simulink model "model"  (R2021a)
settings: Solver=ode23s  StartTime=0.0  StopTime=0.04  MaxStep=1e-4  RelTol=1e-3
undefined symbols (not defined in the file): D1, L, lagging, pulse
libraries: spsACVoltageSourceLib x6, spsSeriesRLCBranchLib x6, spsGroundLib x5, spsThreePhaseTransformerTwoWindingsLib x4, spsUniversalBridgeLib x4, spsVoltageMeasurementLib x3, spsPulseGeneratorThyristor6PulseLib x2, simulink x2, spsControlledCurrentSourceLib x1, spsCurrentMeasurementLib x1, spsPower3phInstantaneousLib x1, spsThreePhaseVIMeasurementLib x1
settings Model: Creator=Tasneem  LastModifiedBy=Tasneem

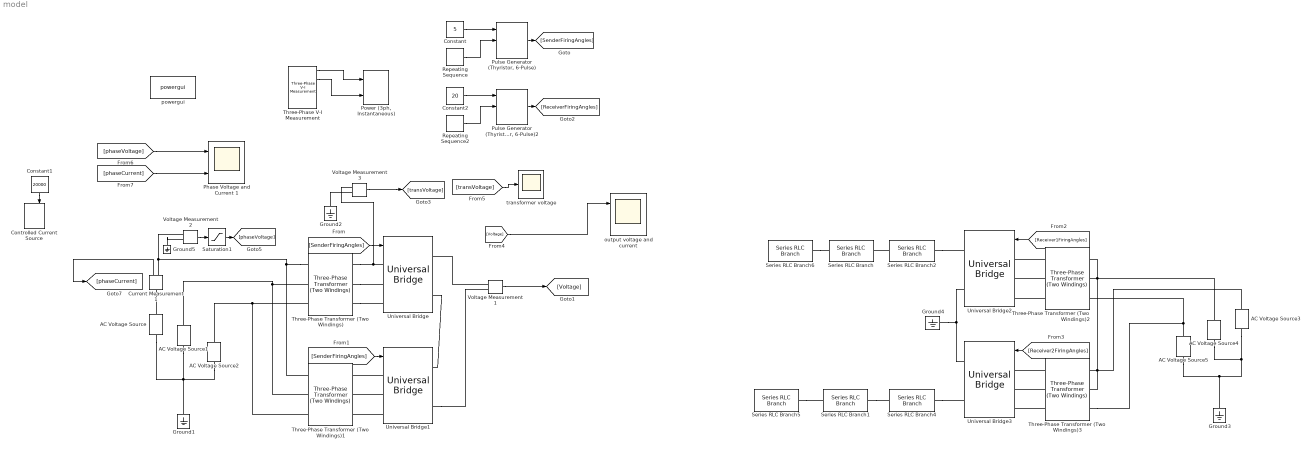
== system model ==
  AC Voltage Source : spsACVoltageSourceLib/AC Voltage Source  Amplitude=22e3  Phase=0  Frequency=50  SampleTime=0  Measurements=None  BusType=swing  Pref=10e3  Qref=0  Qmin=-inf  Qmax=+inf
  AC Voltage Source1 : spsACVoltageSourceLib/AC Voltage Source  Amplitude=22e3  Phase=-120  Frequency=50  SampleTime=0  Measurements=None  BusType=swing  Pref=10e3  Qref=0  Qmin=-inf  Qmax=+inf
  AC Voltage Source2 : spsACVoltageSourceLib/AC Voltage Source  Amplitude=22e3  Phase=120  Frequency=50  SampleTime=0  Measurements=None  BusType=swing  Pref=10e3  Qref=0  Qmin=-inf  Qmax=+inf
  AC Voltage Source3 : spsACVoltageSourceLib/AC Voltage Source  Amplitude=20000*sqrt(2/3)  Phase=0  Frequency=60  SampleTime=0  Measurements=None  BusType=swing  Pref=10e3  Qref=0  Qmin=-inf  Qmax=+inf
  AC Voltage Source4 : spsACVoltageSourceLib/AC Voltage Source  Amplitude=20000*sqrt(2/3)  Phase=-120  Frequency=60  SampleTime=0  Measurements=None  BusType=swing  Pref=10e3  Qref=0  Qmin=-inf  Qmax=+inf
  AC Voltage Source5 : spsACVoltageSourceLib/AC Voltage Source  Amplitude=20000*sqrt(2/3)  Phase=120  Frequency=60  SampleTime=0  Measurements=None  BusType=swing  Pref=10e3  Qref=0  Qmin=-inf  Qmax=+inf
  Constant : Constant  Value=5
  Constant1 : Constant  Value=20000
  Constant2 : Constant  Value=20
  Controlled Current Source : spsControlledCurrentSourceLib/Controlled Current Source  Initialize=on  Source_Type=AC  Amplitude=0  Phase=0  Frequency=0  Measurements=None
  Current Measurement1 : spsCurrentMeasurementLib/Current Measurement  PhasorSimulation=off  OutputType=Complex  PSBequivalent=0
  Ground{1..5} (5 alike) : spsGroundLib/Ground  LConnTagsString=a
  Phase Voltage and Current 1 : Scope  NumInputPorts=2
  "Power (3ph, Instantaneous)" : spsPower3phInstantaneousLib/Power (3ph, Instantaneous)
  "Pulse Generator (Thyristor, 6-Pulse)" : spsPulseGeneratorThyristor6PulseLib/Pulse Generator (Thyristor, 6-Pulse)  GenType=6-pulse  Delta=D1 (lagging)  pwidth=60  Double_Pulse=off  Ts=0
      settings: SourceProductBaseCode=PS
  "Pulse Generator (Thyristor, 6-Pulse)2" : spsPulseGeneratorThyristor6PulseLib/Pulse Generator (Thyristor, 6-Pulse)  GenType=6-pulse  Delta=D1 (lagging)  pwidth=60  Double_Pulse=off  Ts=0
      settings: SourceProductBaseCode=PS
  Repeating Sequence : simulink/Sources/Repeating Sequence  rep_seq_t=[0 1/50]  rep_seq_y=[0 2*pi]
  Repeating Sequence2 : simulink/Sources/Repeating Sequence  rep_seq_t=[0 1/60]  rep_seq_y=[0 2*pi]
  Saturation1 : Saturate  UpperLimit=200e3  LowerLimit=-200e3
  Series RLC Branch : spsSeriesRLCBranchLib/Series RLC Branch  LConnTagsString=__new0  RConnTagsString=__new0  BranchType=R  Resistance=10  Inductance=1e-3  SetiL0=off  InitialCurrent=0  Capacitance=1e-6  Setx0=off  InitialVoltage=0  Measurements=None
  Series RLC Branch1 : spsSeriesRLCBranchLib/Series RLC Branch  LConnTagsString=__new0  RConnTagsString=__new0  BranchType=R  Resistance=10  Inductance=1e-3  SetiL0=off  InitialCurrent=0  Capacitance=1e-6  Setx0=off  InitialVoltage=0  Measurements=None
  Series RLC Branch{2,4..6} (4 alike) : spsSeriesRLCBranchLib/Series RLC Branch  LConnTagsString=__new0  RConnTagsString=__new0  BranchType=L  Resistance=10  Inductance=L  SetiL0=off  InitialCurrent=0  Capacitance=1e-6  Setx0=off  InitialVoltage=0  Measurements=None
  Three-Phase Transformer (Two Windings) : spsThreePhaseTransformerTwoWindingsLib/Three-Phase Transformer (Two Windings)  Winding1Connection=Yg  Winding2Connection=Yg  CoreType=Three single-phase transformers  SetSaturation=off  Hysteresis=off  DataFile='hysteresis'  SetInitialFlux=off  Measurements=None  UNITS=pu  NominalPower=[ 800e6 , 50 ]  Winding1=[ 22e3/sqrt(3) , 0.002 , 0 ]  Winding2=[ 220e3/sqrt(3) , 0.002 , 0 ]  Rm=500  Lm=500  L0=0.49997  Saturation=[ 0,0 ; 0.0024,1.2 ; 1.0,1.52 ]  InitialFluxes=[0.79997 -0.79997 0.69998]  BreakLoop=off  DiscreteSolver=Trapezoidal iterative  DataType=off  TransfoNumber=1
  Three-Phase Transformer (Two Windings)1 : spsThreePhaseTransformerTwoWindingsLib/Three-Phase Transformer (Two Windings)  Winding1Connection=Yg  Winding2Connection=Yg  CoreType=Three single-phase transformers  SetSaturation=off  Hysteresis=off  DataFile='hysteresis'  SetInitialFlux=off  Measurements=None  UNITS=pu  NominalPower=[ 800e6 , 50 ]  Winding1=[ 735e3 , 0.002 , 0 ]  Winding2=[ 20000/sqrt(2) , 0.002 , 0 ]  Rm=500  Lm=500  L0=0.5  Saturation=[ 0,0 ; 0.0024,1.2 ; 1.0,1.52 ]  InitialFluxes=[ 0.8 , -0.8 , 0.7 ]  BreakLoop=off  DiscreteSolver=Trapezoidal iterative  DataType=off  TransfoNumber=1
  Three-Phase Transformer (Two Windings)2 : spsThreePhaseTransformerTwoWindingsLib/Three-Phase Transformer (Two Windings)  Winding1Connection=Yg  Winding2Connection=Yg  CoreType=Three single-phase transformers  SetSaturation=off  Hysteresis=off  DataFile='hysteresis'  SetInitialFlux=off  Measurements=None  UNITS=pu  NominalPower=[ 800e6 , 60 ]  Winding1=[ 20e3/sqrt(3) , 0.002 , 0 ]  Winding2=[ 200e3/sqrt(3) , 0.002 , 0 ]  Rm=500  Lm=500  L0=0.5  Saturation=[ 0,0 ; 0.0024,1.2 ; 1.0,1.52 ]  InitialFluxes=[ 0.8 , -0.8 , 0.7 ]  BreakLoop=off  DiscreteSolver=Trapezoidal iterative  DataType=off  TransfoNumber=1
  Three-Phase Transformer (Two Windings)3 : spsThreePhaseTransformerTwoWindingsLib/Three-Phase Transformer (Two Windings)  Winding1Connection=Yg  Winding2Connection=Yg  CoreType=Three single-phase transformers  SetSaturation=off  Hysteresis=off  DataFile='hysteresis'  SetInitialFlux=off  Measurements=None  UNITS=pu  NominalPower=[ 800e6 , 50 ]  Winding1=[ 735e3 , 0.002 , 0 ]  Winding2=[ 20000/sqrt(2) , 0.002 , 0 ]  Rm=500  Lm=500  L0=0.5  Saturation=[ 0,0 ; 0.0024,1.2 ; 1.0,1.52 ]  InitialFluxes=[ 0.8 , -0.8 , 0.7 ]  BreakLoop=off  DiscreteSolver=Trapezoidal iterative  DataType=off  TransfoNumber=1
  Three-Phase V-I Measurement : spsThreePhaseVIMeasurementLib/Three-Phase V-I Measurement  VoltageMeasurement=phase-to-ground  SetLabelV=off  LabelV=Vabc  Vpu=off  VpuLL=off  CurrentMeasurement=yes  SetLabelI=off  LabelI=Iabc  Ipu=off  Pbase=100e6  Vbase=500e3  OutputType=Complex  PhasorSimulation=off  PSBequivalent=0
  Universal Bridge{,1..3} (4 alike) : spsUniversalBridgeLib/Universal Bridge  Arms=3  SnubberResistance=1e5  SnubberCapacitance=inf  Device=Thyristors  Ron=1e-3  Lon=0  ForwardVoltages="[  0  0  ]"  ForwardVoltage=0  GTOparameters=[ 10e-6 , 20e-6 ]  IGBTparameters=[ 1e-6 , 2e-6 ]  Measurements=None  Measurements_2=None  converterType=Rectifier
  Voltage Measurement1 : spsVoltageMeasurementLib/Voltage Measurement  PhasorSimulation=off  OutputType=Complex  PSBequivalent=0
  Voltage Measurement2 : spsVoltageMeasurementLib/Voltage Measurement  PhasorSimulation=off  OutputType=Complex  PSBequivalent=0
  Voltage Measurement3 : spsVoltageMeasurementLib/Voltage Measurement  PhasorSimulation=off  OutputType=Complex  PSBequivalent=0
  output voltage and current : Scope  NumInputPorts=2
  powergui : spspowerguiLib/powergui  Priority=1  SimulationMode=Discrete  SampleTime=1e-6  frequency=60  Iterations=50  frequencyindice=50  Pbase=100e6  ErrMax=1e-4  UnitsV=kV  UnitsW=MW  buscounter=0  FunctionMessages=off  echomessages=off  EnableUseOfTLC=off  CurrentSourceSwitches=off  DisableSnubberDevices=off  DisableRonSwitches=off  DisableVfSwitches=off  DisplayEquations=off  AutomaticDiscreteSolvers=off  SolverType=Tustin/Backward Euler (TBE)  Interpol=off  ExternalGateDelay=off  methode=off  Ts=100  x0status=blocks  SPID=on  SwTol=0  HookPort=off  NonlinearTolerance=1e-4  nMaxIteration=100  ContinueOnMaxIteration=off  RestoreLinks=warning  ResistiveCurrentMeasurement=off  Frange=[0:2:500]  Ylog=off  Xlog=on  ShowGrid=off  save=off  variable=ZData  structure=0  ZoomFFT=off  StartTime=0.0  cycles=1  DisplayStyle=1  fundamental=60  FreqAxis=off  MaxFrequency=1000  frequencyindicesteady=1  RmsSteady=1  display=off
  transformer voltage : Scope
  wires:
  Constant/1 -> "Pulse Generator (Thyristor, 6-Pulse)"/1
  Repeating Sequence/1 -> "Pulse Generator (Thyristor, 6-Pulse)"/2
  Three-Phase V-I Measurement/1 -> "Power (3ph, Instantaneous)"/1
  Three-Phase V-I Measurement/2 -> "Power (3ph, Instantaneous)"/2
  [SenderFiringAngles] -> Universal Bridge/1
  "Pulse Generator (Thyristor, 6-Pulse)"/1 -> [SenderFiringAngles]
  [SenderFiringAngles] -> Universal Bridge1/1
  [Receiver2FiringAngles] -> Universal Bridge3/1
  [Receiver1FiringAngles] -> Universal Bridge2/1
  "Pulse Generator (Thyristor, 6-Pulse)2"/1 -> [ReceiverFiringAngles]
  Repeating Sequence2/1 -> "Pulse Generator (Thyristor, 6-Pulse)2"/2
  Constant2/1 -> "Pulse Generator (Thyristor, 6-Pulse)2"/1
  Current Measurement1/1 -> [phaseCurrent]
  [phaseCurrent] -> Phase Voltage and Current 1/2
  [phaseVoltage] -> Phase Voltage and Current 1/1
  Voltage Measurement2/1 -> Saturation1/1
  Saturation1/1 -> [phaseVoltage]
  Voltage Measurement1/1 -> [Voltage]
  [Voltage] -> output voltage and current/1
  Constant1/1 -> Controlled Current Source/1
  Voltage Measurement3/1 -> [transVoltage]
  [transVoltage] -> transformer voltage/1
  connections:
  AC Voltage Source/LConn1 -- Ground1/LConn1 -- AC Voltage Source2/LConn1 -- AC Voltage Source1/LConn1
  Three-Phase Transformer (Two Windings)/LConn1 -- Current Measurement1/RConn1 -- Voltage Measurement2/LConn1 -- Three-Phase Transformer (Two Windings)1/LConn1
  AC Voltage Source1/RConn1 -- Three-Phase Transformer (Two Windings)1/LConn2 -- Three-Phase Transformer (Two Windings)/LConn2
  AC Voltage Source2/RConn1 -- Three-Phase Transformer (Two Windings)1/LConn3 -- Three-Phase Transformer (Two Windings)/LConn3
  Three-Phase Transformer (Two Windings)/RConn2 -- Universal Bridge/LConn2
  Three-Phase Transformer (Two Windings)/RConn1 -- Voltage Measurement3/LConn1 -- Universal Bridge/LConn1
  Three-Phase Transformer (Two Windings)/RConn3 -- Universal Bridge/LConn3
  Universal Bridge1/LConn1 -- Three-Phase Transformer (Two Windings)1/RConn1
  Universal Bridge1/LConn2 -- Three-Phase Transformer (Two Windings)1/RConn2
  Universal Bridge1/LConn3 -- Three-Phase Transformer (Two Windings)1/RConn3
  AC Voltage Source3/LConn1 -- AC Voltage Source5/LConn1 -- Ground3/LConn1 -- AC Voltage Source4/LConn1
  AC Voltage Source3/RConn1 -- Three-Phase Transformer (Two Windings)2/LConn1 -- Three-Phase Transformer (Two Windings)3/LConn1
  AC Voltage Source4/RConn1 -- Three-Phase Transformer (Two Windings)2/LConn2 -- Three-Phase Transformer (Two Windings)3/LConn2
  Three-Phase Transformer (Two Windings)3/LConn3 -- AC Voltage Source5/RConn1 -- Three-Phase Transformer (Two Windings)2/LConn3
  Universal Bridge2/RConn2 -- Ground4/LConn1 -- Universal Bridge3/RConn1
  Three-Phase Transformer (Two Windings)3/RConn3 -- Universal Bridge3/LConn3
  Three-Phase Transformer (Two Windings)3/RConn2 -- Universal Bridge3/LConn2
  Three-Phase Transformer (Two Windings)3/RConn1 -- Universal Bridge3/LConn1
  Three-Phase Transformer (Two Windings)2/RConn2 -- Universal Bridge2/LConn2
  Three-Phase Transformer (Two Windings)2/RConn1 -- Universal Bridge2/LConn1
  Three-Phase Transformer (Two Windings)2/RConn3 -- Universal Bridge2/LConn3
  Series RLC Branch2/LConn1 -- Series RLC Branch/RConn1
  Series RLC Branch4/RConn1 -- Universal Bridge3/RConn2
  Series RLC Branch2/RConn1 -- Universal Bridge2/RConn1
  Series RLC Branch5/RConn1 -- Series RLC Branch1/LConn1
  Series RLC Branch1/RConn1 -- Series RLC Branch4/LConn1
  Ground5/LConn1 -- Voltage Measurement2/LConn2
  AC Voltage Source/RConn1 -- Current Measurement1/LConn1
  Series RLC Branch6/RConn1 -- Series RLC Branch/LConn1
  Voltage Measurement1/LConn1 -- Universal Bridge/RConn1
  Voltage Measurement3/LConn2 -- Ground2/LConn1
  Universal Bridge/RConn2 -- Universal Bridge1/RConn1
  Universal Bridge1/RConn2 -- Voltage Measurement1/LConn2
